simulink model "P5e"  (Simulink 8.5)
settings: Solver=ode45  StartTime=0.0  StopTime=500  RelTol=1e-3
values from neighbouring files (symbols this model uses):
  psi_ref = 30    [Part_5.m]    (also in p5p5c_script.m; p5p5d_script.m; p5p5e_script.m)
  Ts = 0.1    [Part_5.m]    (also in p5p5c_script.m)
undefined symbols (not defined in the file or in its folder): K_pd, T_d, T_f
libraries: simulink x2
settings Model: Creator=markh  LastModifiedBy=bendikss
settings DataIOCC: InitialState=x0  SignalLoggingName=sigsOut
settings OptimizationCC: ExpressionDepthLimit=128  InitFltsAndDblsToZero=on
settings DebuggingCC: SaveWithParameterizedLinksMsg=none  SignalResolutionControl=TryResolveAllWithWarning  MultiTaskDSMMsg=warning  MultiTaskCondExecSysMsg=none  FcnCallInpInsideContextMsg=UseLocalSettings
settings HardwareCC: TargetUnknown=on
settings GRTTargetCC: TargetFcnLib=ansi_tfl_tmw.mat

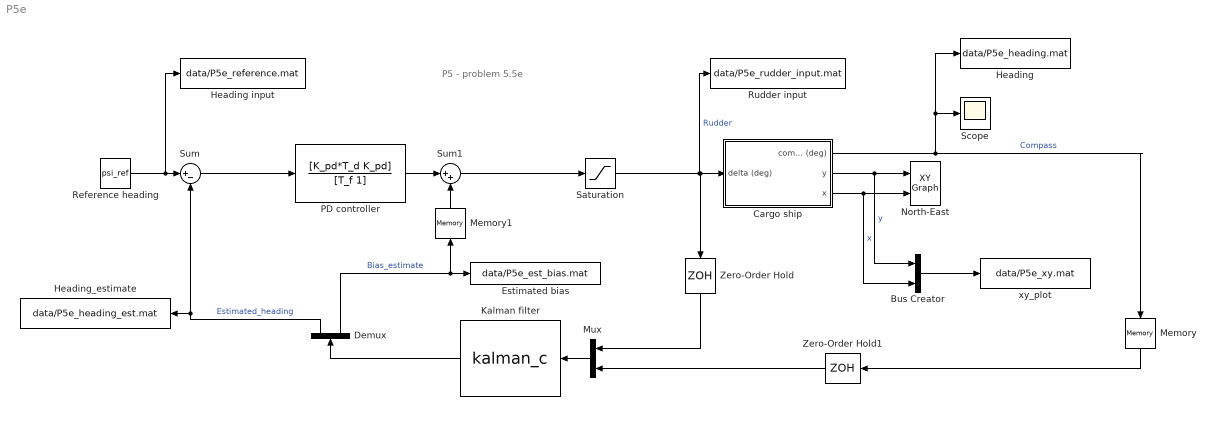
== system P5e ==
  note: P5 - problem 5.5e
  Bus Creator : BusCreator  Inputs=2
  Cargo ship : Subsystem  mask(Simple shipmodel for a cargo ship){noise=on, current=on, logic=on}
      mask prompts: noise "measurement noise"; logic "waves"
      mask help:
      | Measurement noise:
      | 	checked = noise on
      | 	unchecked = noise off
      |
      | Current:
      | 	checked = current on
      | 	unchecked = current off
      |
      | Waves:
      | 	checked = waves on
      | 	unchecked = waves off
      |
      | Author: Jørgen Spjøtvold, 9/10-2003
      | TTK 4115 Linear system theory.
      | Modified by Jostein Bakkeheim 26/10-2006
  Demux : Demux  Outputs=2
  Estimated bias : ToFile  Filename=data/P5e_est_bias.mat  MatrixName=est_bias_5e  SaveFormat=Timeseries
  Heading : ToFile  Filename=data/P5e_heading.mat  MatrixName=heading_5e  SaveFormat=Timeseries
  Heading input : ToFile  Filename=data/P5e_reference.mat  MatrixName=heading_reference_5e  SaveFormat=Timeseries
  Heading_estimate : ToFile  Filename=data/P5e_heading_est.mat  MatrixName=est_heading_5e  SaveFormat=Timeseries
  Kalman filter : S-Function  FunctionName=kalman_c  Parameters=sys  SFunctionModules=part5
  Memory : Memory
  Memory1 : Memory
  Mux : Mux  Inputs=2
  North-East : simulink/Sinks/XY Graph  xmin=-5000  xmax=5000  ymin=-5000  ymax=5000  st=-1
  PD controller : TransferFcn  Numerator=[K_pd*T_d K_pd]  Denominator=[T_f 1]  ContinuousStateAttributes='Heading'
  Reference heading : Constant  Value=psi_ref
  Rudder input : ToFile  Filename=data/P5e_rudder_input.mat  MatrixName=rudder_input_5e  SaveFormat=Timeseries
  Saturation : Saturate  UpperLimit=35  LowerLimit=-35
  Scope : Scope
      settings: YMin=26.5  YMax=32.25
  Sum : Sum  Inputs=|+-
  Sum1 : Sum  Inputs=|++
  Zero-Order Hold : ZeroOrderHold  SampleTime=Ts
  Zero-Order Hold1 : ZeroOrderHold  SampleTime=Ts
  xy_plot : ToFile  Filename=data/P5e_xy.mat  MatrixName=xy_plot_5e  SaveFormat=Timeseries
  wires:
  Cargo ship/3(x) -> Bus Creator/2, North-East/2  "x"
  Cargo ship/2(y) -> Bus Creator/1, North-East/1  "y"
  Cargo ship/1(compass (deg)) -> Scope/1, Heading/1, Memory/1  "Compass"
  Reference heading/1 -> Heading input/1, Sum/1
  Sum/1 -> PD controller/1
  Saturation/1 -> Zero-Order Hold/1, Cargo ship/1(delta (deg)), Rudder input/1  "Rudder"
  Bus Creator/1 -> xy_plot/1
  Mux/1 -> Kalman filter/1
  Zero-Order Hold1/1 -> Mux/2
  Zero-Order Hold/1 -> Mux/1
  PD controller/1 -> Sum1/1
  Sum1/1 -> Saturation/1
  Kalman filter/1 -> Demux/1
  Demux/2 -> Memory1/1, Estimated bias/1  "Bias_estimate"
  Memory/1 -> Zero-Order Hold1/1
  Memory1/1 -> Sum1/2
  Demux/1 -> Heading_estimate/1, Sum/2  "Estimated_heading"

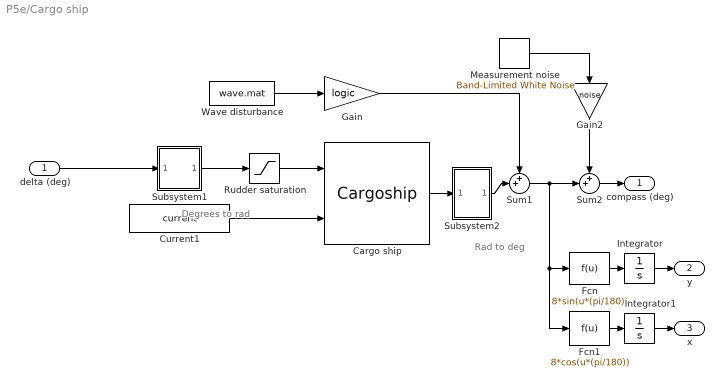
== system P5e/Cargo ship ==
  note: Degrees to rad
  note: Rad to deg
  delta (deg) : Inport
  Cargo ship : S-Function  FunctionName=Cargoship  mask(Cargo ship){}
      mask help:
      | S-function which simulates a cargo ship.
      |
      | Author: Jørgen Spjøtvold
      | 20.10-2003
      | Modified by Jostein Bakkeheim 27.10.2006
  Current1 : Constant  Value=current
  Fcn : Fcn  Expr=8*sin(u*(pi/180))
  Fcn1 : Fcn  Expr=8*cos(u*(pi/180))
  Gain : Gain  Gain=logic  SaturateOnIntegerOverflow=on  OutDataTypeStr=Inherit: Same as input  ParamDataTypeStr=Inherit: Same as input
  Gain2 : Gain  Gain=noise  SaturateOnIntegerOverflow=on  OutDataTypeStr=Inherit: Same as input  ParamDataTypeStr=Inherit: Same as input
  Integrator : Integrator
  Integrator1 : Integrator
  Measurement noise : simulink/Sources/Band-Limited White Noise  Cov=[0.001]  Ts=.5  seed=[23341]
  Rudder saturation : Saturate  UpperLimit=45*(pi/180)  LowerLimit=-45*(pi/180)
  Subsystem1 : Subsystem  mask(degrees to radians){}
      mask help: Converts degrees to radians
      mask Display: fprintf('D2R');
  Subsystem2 : Subsystem  mask(radians to degrees){}
      mask help: Converts radians to degrees
      mask Display: fprintf('R2D');
  Sum1 : Sum  Inputs=++|  SaturateOnIntegerOverflow=on
  Sum2 : Sum  Inputs=++|  SaturateOnIntegerOverflow=on
  Wave disturbance : FromFile  FileName=wave.mat  SampleTime=0
  compass (deg) : Outport
  y : Outport  Port=2
  x : Outport  Port=3
  wires:
  delta (deg)/1 -> Subsystem1/1(In1)
  Fcn/1 -> Integrator/1
  Integrator/1 -> y/1
  Fcn1/1 -> Integrator1/1
  Integrator1/1 -> x/1
  Wave disturbance/1 -> Gain/1
  Subsystem2/1(Out1) -> Sum1/2
  Gain/1 -> Sum1/1
  Sum1/1 -> Fcn/1, Fcn1/1, Sum2/2
  Cargo ship/1 -> Subsystem2/1(In1)
  Subsystem1/1(Out1) -> Rudder saturation/1
  Rudder saturation/1 -> Cargo ship/1
  Sum2/1 -> compass (deg)/1
  Measurement noise/1 -> Gain2/1
  Gain2/1 -> Sum2/1
  Current1/1 -> Cargo ship/2

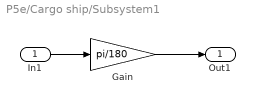
== system P5e/Cargo ship/Subsystem1 ==
  In1 : Inport
  Gain : Gain  Gain=pi/180  SaturateOnIntegerOverflow=on  OutDataTypeStr=Inherit: Same as input  ParamDataTypeStr=Inherit: Same as input
  Out1 : Outport
  wires:
  Gain/1 -> Out1/1
  In1/1 -> Gain/1

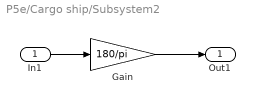
== system P5e/Cargo ship/Subsystem2 ==
  In1 : Inport
  Gain : Gain  Gain=180/pi  SaturateOnIntegerOverflow=on  OutDataTypeStr=Inherit: Same as input  ParamDataTypeStr=Inherit: Same as input
  Out1 : Outport
  wires:
  Gain/1 -> Out1/1
  In1/1 -> Gain/1
